simulink model "state_feedback_simulink"  (R2015b)
settings: Solver=ode3  StartTime=0.0  StopTime=10  FixedStep=0.01  RelTol=1e-3
values from neighbouring files (symbols this model uses):
  K = place(A,B,P)    [drone_config.m]
libraries: aerolib6dof2 x1
settings Model: Creator=rcasado  LastModifiedBy=rcasado
settings DataIOCC: SaveFormat=Array
settings DebuggingCC: MultiTaskRateTransMsg=warning
settings HardwareCC: ProdBitPerPointer=32  ProdLargestAtomicFloat=None  ProdIntDivRoundTo=Undefined  ProdEndianess=Unspecified  ProdWordSize=32  ProdHWDeviceType=32-bit Generic
settings GRTTargetCC: GeneratePreprocessorConditionals=Disable all
settings ConfigComp: CovModelRefEnable=Off

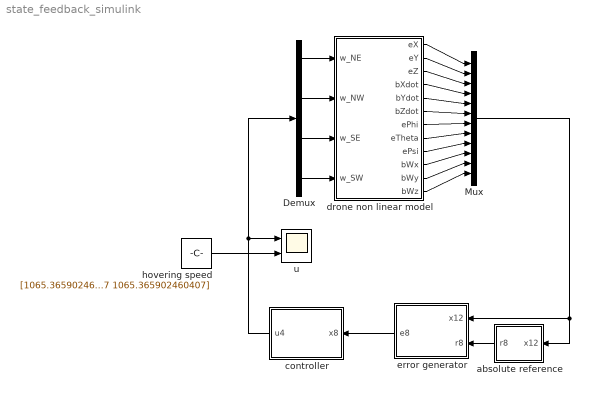
== system state_feedback_simulink ==
  Demux : Demux
  Mux : Mux  Inputs=12
  absolute reference : Subsystem
  controller : Subsystem
  drone non linear model : Subsystem
  error generator : Subsystem
  hovering speed : Constant  Value=[1065.365902460407 1065.365902460407 1065.365902460407 1065.365902460407]
  u : Scope  NumInputPorts=2
  wires:
  drone non linear model/1(eX) -> Mux/1
  drone non linear model/3(eZ) -> Mux/3
  drone non linear model/2(eY) -> Mux/2
  Demux/1 -> drone non linear model/1(w_NE)
  Demux/2 -> drone non linear model/2(w_NW)
  Demux/3 -> drone non linear model/3(w_SE)
  Demux/4 -> drone non linear model/4(w_SW)
  drone non linear model/12(bWz) -> Mux/12
  drone non linear model/11(bWy) -> Mux/11
  drone non linear model/4(bXdot) -> Mux/4
  drone non linear model/5(bYdot) -> Mux/5
  drone non linear model/6(bZdot) -> Mux/6
  drone non linear model/7(ePhi) -> Mux/7
  drone non linear model/8(eTheta) -> Mux/8
  drone non linear model/9(ePsi) -> Mux/9
  drone non linear model/10(bWx) -> Mux/10
  hovering speed/1 -> u/2
  Mux/1 -> absolute reference/1(x12), error generator/1(x12)
  error generator/1(e8) -> controller/1(x8)
  absolute reference/1(r8) -> error generator/2(r8)
  controller/1(u4) -> Demux/1, u/1

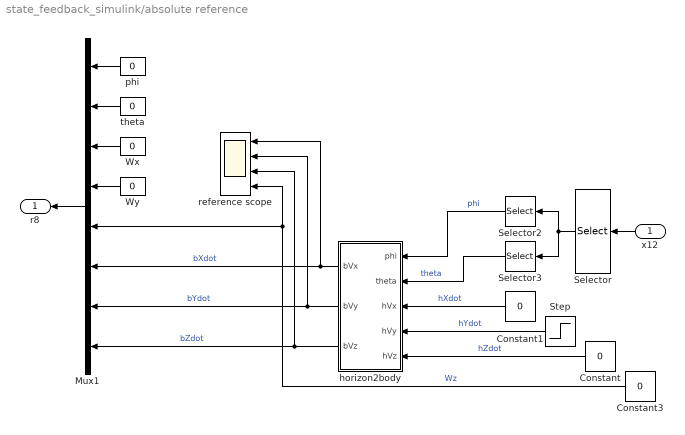
== system state_feedback_simulink/absolute reference ==
  x12 : Inport
  Constant : Constant  Value=0
  Constant1 : Constant  Value=0
  Constant3 : Constant  Value=0
  Mux1 : Mux  Inputs=8
  Selector : Selector  InputPortWidth=12  IndexOptions=Index vector (dialog)  Indices=[7,8]  OutputSizes=1
  Selector2 : Selector  InputPortWidth=2  IndexOptions=Index vector (dialog)  Indices=[1]  OutputSizes=1
  Selector3 : Selector  InputPortWidth=2  IndexOptions=Index vector (dialog)  Indices=[2]  OutputSizes=1
  Step : Step  Time=2  After=2  SampleTime=0
  Wx : Constant  Value=0
  Wy : Constant  Value=0
  horizon2body : Subsystem
  phi : Constant  Value=0
  reference scope : Scope  NumInputPorts=4
  theta : Constant  Value=0
  r8 : Outport
  wires:
  Step/1 -> horizon2body/4(hVy)  "hYdot"
  Constant1/1 -> horizon2body/3(hVx)  "hXdot"
  Constant3/1 -> Mux1/5, reference scope/4  "Wz"
  Constant/1 -> horizon2body/5(hVz)  "hZdot"
  Selector2/1 -> horizon2body/1(phi)  "phi"
  Selector3/1 -> horizon2body/2(theta)  "theta"
  x12/1 -> Selector/1
  Selector/1 -> Selector2/1, Selector3/1
  Mux1/1 -> r8/1
  Wx/1 -> Mux1/3
  Wy/1 -> Mux1/4
  horizon2body/1(bVx) -> reference scope/1, Mux1/6  "bXdot"
  horizon2body/3(bVz) -> Mux1/8, reference scope/3  "bZdot"
  horizon2body/2(bVy) -> reference scope/2, Mux1/7  "bYdot"
  phi/1 -> Mux1/1
  theta/1 -> Mux1/2

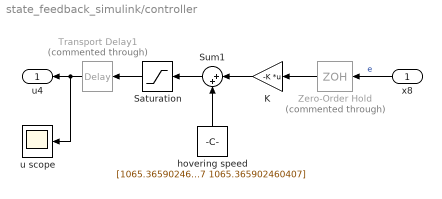
== system state_feedback_simulink/controller ==
  x8 : Inport
  K : Gain  Gain=-K  Multiplication=Matrix(K*u)
  Saturation : Saturate  UpperLimit=1650  LowerLimit=0
  Sum1 : Sum  Inputs=|++
  Transport Delay1 : TransportDelay  Commented=through  DelayTime=0.05
  Zero-Order Hold : ZeroOrderHold  Commented=through  SampleTime=0.01
  hovering speed : Constant  Value=[1065.365902460407 1065.365902460407 1065.365902460407 1065.365902460407]
  u scope : Scope
  u4 : Outport
  wires:
  Saturation/1 -> Transport Delay1/1
  K/1 -> Sum1/1
  x8/1 -> Zero-Order Hold/1  "e"
  hovering speed/1 -> Sum1/2
  Sum1/1 -> Saturation/1
  Zero-Order Hold/1 -> K/1
  Transport Delay1/1 -> u scope/1, u4/1

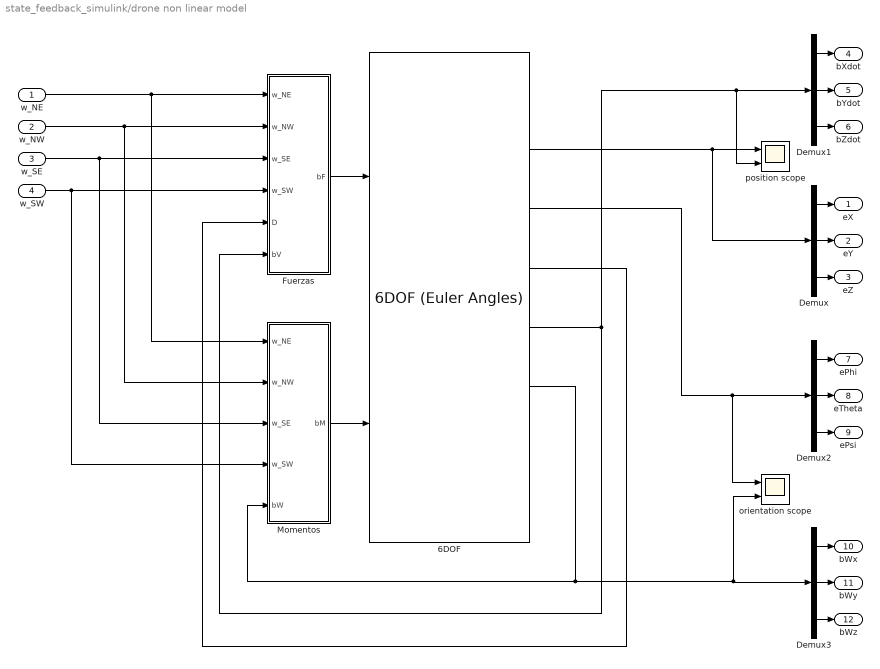
== system state_feedback_simulink/drone non linear model ==
  w_NE : Inport
  w_NW : Inport  Port=2
  w_SE : Inport  Port=3
  w_SW : Inport  Port=4
  6DOF : aerolib6dof2/6DOF (Euler Angles)  units=Metric (MKS)  mtype=Fixed  rep=Euler Angles  xme_0=[0 0 10]  Vm_0=[0 0 0]  eul_0=[0 0 deg2rad(0)]  pm_0=[0 0 0]  mass_0=1.840  mass_e=0.5  mass_f=2.0  inertia="[0.024916667  0  0 ; 0 0.024916667 0 ; 0 0 0.049066667]"  inertia_e=eye(3)  inertia_f=2*eye(3)  k_quat=1.0  vre_flag=on
  Demux{,1..3} (4 alike) : Demux  Outputs=3
  Fuerzas : Subsystem
  Momentos : Subsystem
  orientation scope : Scope  NumInputPorts=2
  position scope : Scope  NumInputPorts=2
  eX : Outport
  eY : Outport  Port=2
  eZ : Outport  Port=3
  bXdot : Outport  Port=4
  bYdot : Outport  Port=5
  bZdot : Outport  Port=6
  ePhi : Outport  Port=7
  eTheta : Outport  Port=8
  ePsi : Outport  Port=9
  bWx : Outport  Port=10
  bWy : Outport  Port=11
  bWz : Outport  Port=12
  wires:
  6DOF/2 -> Demux/1, position scope/1
  Momentos/1(bM) -> 6DOF/2
  w_NE/1 -> Momentos/1(w_NE), Fuerzas/1(w_NE)
  w_NW/1 -> Momentos/2(w_NW), Fuerzas/2(w_NW)
  w_SE/1 -> Momentos/3(w_SE), Fuerzas/3(w_SE)
  w_SW/1 -> Momentos/4(w_SW), Fuerzas/4(w_SW)
  6DOF/4 -> Fuerzas/5(D)
  Fuerzas/1(bF) -> 6DOF/1
  6DOF/6 -> Demux3/1, orientation scope/2, Momentos/5(bW)
  Demux/1 -> eX/1
  Demux/2 -> eY/1
  Demux/3 -> eZ/1
  6DOF/5 -> position scope/2, Demux1/1, Fuerzas/6(bV)
  Demux1/1 -> bXdot/1
  Demux1/2 -> bYdot/1
  Demux1/3 -> bZdot/1
  Demux2/1 -> ePhi/1
  Demux2/2 -> eTheta/1
  Demux2/3 -> ePsi/1
  Demux3/1 -> bWx/1
  Demux3/2 -> bWy/1
  Demux3/3 -> bWz/1
  6DOF/3 -> orientation scope/1, Demux2/1

== system state_feedback_simulink/error generator ==
  x12 : Inport
  r8 : Inport  Port=2
  Selector : Selector  InputPortWidth=12  IndexOptions=Index vector (dialog)  Indices=[7 8 10 11 12 4 5 6]  OutputSizes=1
  Sum : Sum  Inputs=|+-
  error scope : Scope
  estado scope : Scope
  referencia scope : Scope
  e8 : Outport
  wires:
  Sum/1 -> e8/1, error scope/1
  Selector/1 -> estado scope/1, Sum/1
  r8/1 -> Sum/2, referencia scope/1
  x12/1 -> Selector/1

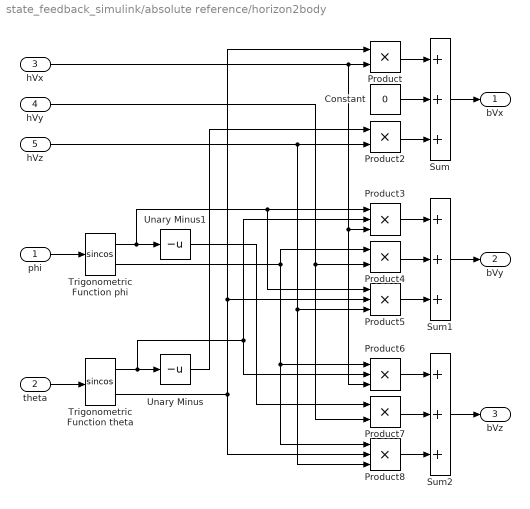
== system state_feedback_simulink/absolute reference/horizon2body ==
  phi : Inport
  theta : Inport  Port=2
  hVx : Inport  Port=3
  hVy : Inport  Port=4
  hVz : Inport  Port=5
  Constant : Constant  Value=0
  Product{,2,4,7} (4 alike) : Product
  Product{3,5..6,8} (4 alike) : Product  Inputs=3
  Sum : Sum  Inputs=3
  Sum1 : Sum  Inputs=3
  Sum2 : Sum  Inputs=3
  Trigonometric Function phi : Trigonometry  Operator=sincos
  Trigonometric Function theta : Trigonometry  Operator=sincos
  Unary Minus : UnaryMinus
  Unary Minus1 : UnaryMinus
  bVx : Outport
  bVy : Outport  Port=2
  bVz : Outport  Port=3
  wires:
  theta/1 -> Trigonometric Function theta/1
  phi/1 -> Trigonometric Function phi/1
  Trigonometric Function phi/2 -> Product4/1, Product8/1, Product6/1
  Trigonometric Function theta/2 -> Product8/2, Product/1, Product5/2
  Trigonometric Function theta/1 -> Product3/2, Product6/2, Unary Minus/1
  Trigonometric Function phi/1 -> Unary Minus1/1, Product5/1, Product3/1
  Sum/1 -> bVx/1
  Sum1/1 -> bVy/1
  Sum2/1 -> bVz/1
  Product/1 -> Sum/1
  Constant/1 -> Sum/2
  Product2/1 -> Sum/3
  Product3/1 -> Sum1/1
  Product4/1 -> Sum1/2
  Product5/1 -> Sum1/3
  Product6/1 -> Sum2/1
  Product7/1 -> Sum2/2
  Product8/1 -> Sum2/3
  hVx/1 -> Product6/3, Product3/3, Product/2
  hVy/1 -> Product7/2, Product4/2
  hVz/1 -> Product8/3, Product5/3, Product2/2
  Unary Minus/1 -> Product2/1
  Unary Minus1/1 -> Product7/1

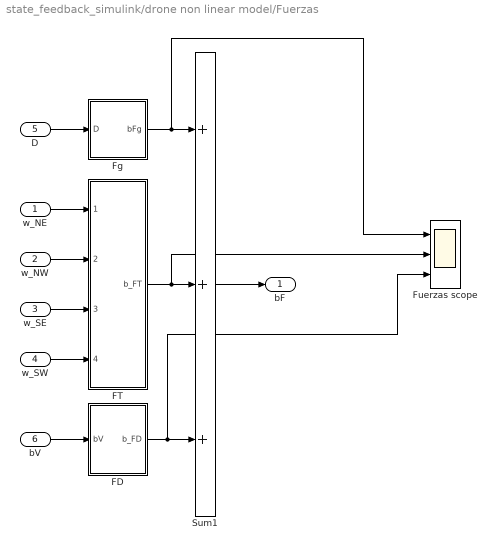
== system state_feedback_simulink/drone non linear model/Fuerzas ==
  w_NE : Inport
  w_NW : Inport  Port=2
  w_SE : Inport  Port=3
  w_SW : Inport  Port=4
  D : Inport  Port=5
  bV : Inport  Port=6
  FD : Subsystem
  FT : Subsystem
  Fg : Subsystem
  Fuerzas scope : Scope  NumInputPorts=3
  Sum1 : Sum  Inputs=+++
  bF : Outport
  wires:
  D/1 -> Fg/1(D)
  Fg/1(bFg) -> Fuerzas scope/1, Sum1/1
  FT/1(b_FT) -> Fuerzas scope/2, Sum1/2
  w_SW/1 -> FT/4(w_SW)
  w_NE/1 -> FT/1(w_NE)
  w_SE/1 -> FT/3(w_SE)
  w_NW/1 -> FT/2(w_NW)
  Sum1/1 -> bF/1
  bV/1 -> FD/1(bV)
  FD/1(b_FD) -> Sum1/3, Fuerzas scope/3

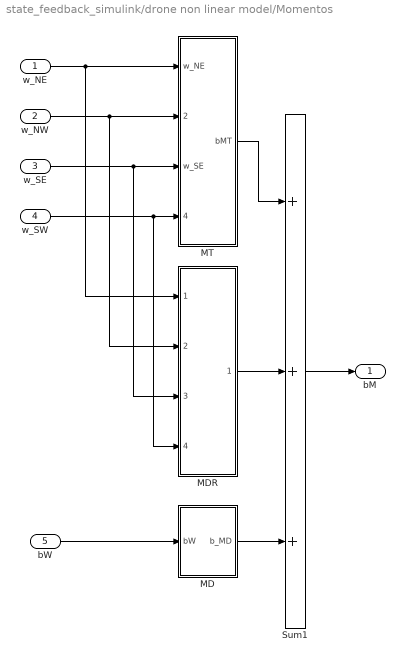
== system state_feedback_simulink/drone non linear model/Momentos ==
  w_NE : Inport
  w_NW : Inport  Port=2
  w_SE : Inport  Port=3
  w_SW : Inport  Port=4
  bW : Inport  Port=5
  MD : Subsystem
  MDR : Subsystem
  MT : Subsystem
  Sum1 : Sum  Inputs=+++
  bM : Outport
  wires:
  bW/1 -> MD/1(bW)
  MT/1(bMT) -> Sum1/1
  w_SW/1 -> MDR/4(w_SW), MT/4(w_SW)
  w_NE/1 -> MDR/1(w_NE), MT/1(w_NE)
  w_SE/1 -> MDR/3(w_SE), MT/3(w_SE)
  w_NW/1 -> MDR/2(w_NW), MT/2(w_NW)
  Sum1/1 -> bM/1
  MD/1(b_MD) -> Sum1/3
  MDR/1(b_MDR) -> Sum1/2

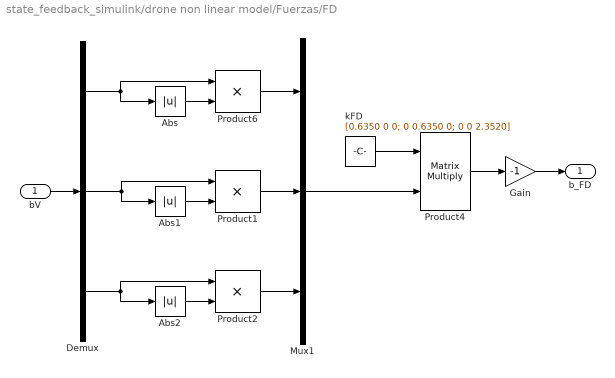
== system state_feedback_simulink/drone non linear model/Fuerzas/FD ==
  bV : Inport
  Abs : Abs
  Abs1 : Abs
  Abs2 : Abs
  Demux : Demux  Outputs=3
  Gain : Gain  Gain=-1
  Mux1 : Mux  Inputs=3
  Product1 : Product
  Product2 : Product
  Product4 : Product  Multiplication=Matrix(*)
  Product6 : Product
  kFD : Constant  Value=[0.6350 0 0; 0 0.6350 0; 0 0 2.3520]
  b_FD : Outport
  wires:
  kFD/1 -> Product4/1
  Product4/1 -> Gain/1
  Mux1/1 -> Product4/2
  Product1/1 -> Mux1/2
  bV/1 -> Demux/1
  Abs/1 -> Product6/2
  Abs1/1 -> Product1/2
  Abs2/1 -> Product2/2
  Demux/1 -> Product6/1, Abs/1
  Demux/2 -> Product1/1, Abs1/1
  Demux/3 -> Product2/1, Abs2/1
  Product6/1 -> Mux1/1
  Product2/1 -> Mux1/3
  Gain/1 -> b_FD/1

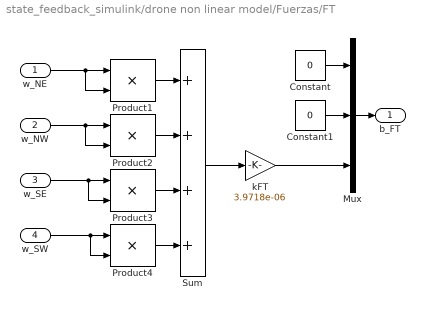
== system state_feedback_simulink/drone non linear model/Fuerzas/FT ==
  w_NE : Inport
  w_NW : Inport  Port=2
  w_SE : Inport  Port=3
  w_SW : Inport  Port=4
  Constant : Constant  Value=0
  Constant1 : Constant  Value=0
  Mux : Mux  Inputs=3
  Product{1..4} (4 alike) : Product
  Sum : Sum  Inputs=++++
  kFT : Gain  Gain=3.9718e-06
  b_FT : Outport
  wires:
  Product4/1 -> Sum/4
  Product3/1 -> Sum/3
  Product2/1 -> Sum/2
  w_NW/1 -> Product2/2, Product2/1
  w_NE/1 -> Product1/2, Product1/1
  Product1/1 -> Sum/1
  Mux/1 -> b_FT/1
  w_SE/1 -> Product3/2, Product3/1
  w_SW/1 -> Product4/2, Product4/1
  Sum/1 -> kFT/1
  Constant/1 -> Mux/1
  Constant1/1 -> Mux/2
  kFT/1 -> Mux/3

== system state_feedback_simulink/drone non linear model/Fuerzas/Fg ==
  D : Inport
  Fg scope : Scope  Commented=on  NumInputPorts=2
  Product : Product  Multiplication=Matrix(*)
  g : Gain  Gain=[0; 0; -9.8]
  masa : Constant  Value=1.840
  bFg : Outport
  wires:
  Product/1 -> Fg scope/2, bFg/1
  D/1 -> Product/1
  masa/1 -> g/1
  g/1 -> Fg scope/1, Product/2  "Fg"

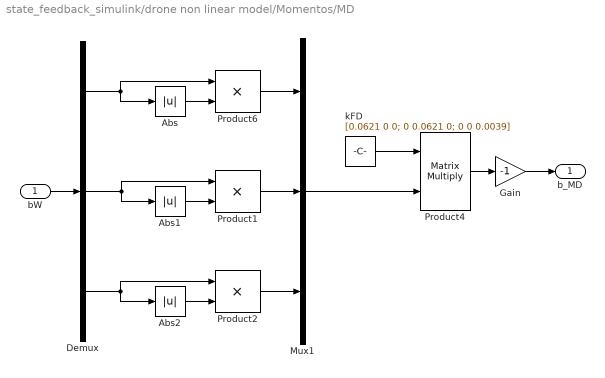
== system state_feedback_simulink/drone non linear model/Momentos/MD ==
  bW : Inport
  Abs : Abs
  Abs1 : Abs
  Abs2 : Abs
  Demux : Demux  Outputs=3
  Gain : Gain  Gain=-1
  Mux1 : Mux  Inputs=3
  Product1 : Product
  Product2 : Product
  Product4 : Product  Multiplication=Matrix(*)
  Product6 : Product
  kFD : Constant  Value=[0.0621 0 0; 0 0.0621 0; 0 0 0.0039]
  b_MD : Outport
  wires:
  kFD/1 -> Product4/1
  Product4/1 -> Gain/1
  Mux1/1 -> Product4/2
  Product1/1 -> Mux1/2
  bW/1 -> Demux/1
  Abs/1 -> Product6/2
  Abs1/1 -> Product1/2
  Abs2/1 -> Product2/2
  Demux/1 -> Product6/1, Abs/1
  Demux/2 -> Product1/1, Abs1/1
  Demux/3 -> Product2/1, Abs2/1
  Product6/1 -> Mux1/1
  Product2/1 -> Mux1/3
  Gain/1 -> b_MD/1

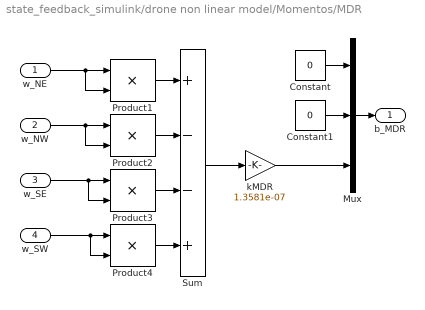
== system state_feedback_simulink/drone non linear model/Momentos/MDR ==
  w_NE : Inport
  w_NW : Inport  Port=2
  w_SE : Inport  Port=3
  w_SW : Inport  Port=4
  Constant : Constant  Value=0
  Constant1 : Constant  Value=0
  Mux : Mux  Inputs=3
  Product{1..4} (4 alike) : Product
  Sum : Sum  Inputs=+--+
  kMDR : Gain  Gain=1.3581e-07
  b_MDR : Outport
  wires:
  Product4/1 -> Sum/4
  Product3/1 -> Sum/3
  Product2/1 -> Sum/2
  w_NW/1 -> Product2/2, Product2/1
  w_NE/1 -> Product1/2, Product1/1
  Product1/1 -> Sum/1
  Mux/1 -> b_MDR/1
  w_SE/1 -> Product3/2, Product3/1
  w_SW/1 -> Product4/2, Product4/1
  Sum/1 -> kMDR/1
  Constant/1 -> Mux/1
  Constant1/1 -> Mux/2
  kMDR/1 -> Mux/3

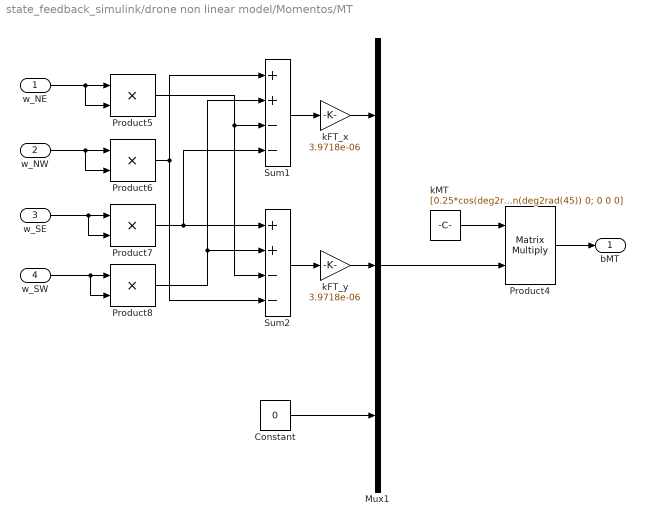
== system state_feedback_simulink/drone non linear model/Momentos/MT ==
  w_NE : Inport
  w_NW : Inport  Port=2
  w_SE : Inport  Port=3
  w_SW : Inport  Port=4
  Constant : Constant  Value=0
  Mux1 : Mux  Inputs=3
  Product4 : Product  Multiplication=Matrix(*)
  Product{5..8} (4 alike) : Product
  Sum1 : Sum  Inputs=++--
  Sum2 : Sum  Inputs=++--
  kFT_x : Gain  Gain=3.9718e-06
  kFT_y : Gain  Gain=3.9718e-06
  kMT : Constant  Value=[0.25*cos(deg2rad(45)) 0 0; 0 0.25*sin(deg2rad(45)) 0; 0 0 0]
  bMT : Outport
  wires:
  kMT/1 -> Product4/1
  Product4/1 -> bMT/1
  Product8/1 -> Sum1/2, Sum2/2
  Product7/1 -> Sum2/1, Sum1/4
  w_NW/1 -> Product6/2, Product6/1
  w_NE/1 -> Product5/2, Product5/1
  Product6/1 -> Sum2/4, Sum1/1
  Mux1/1 -> Product4/2
  w_SE/1 -> Product7/2, Product7/1
  w_SW/1 -> Product8/2, Product8/1
  kFT_y/1 -> Mux1/2
  Sum1/1 -> kFT_x/1
  Sum2/1 -> kFT_y/1
  Product5/1 -> Sum2/3, Sum1/3
  kFT_x/1 -> Mux1/1
  Constant/1 -> Mux1/3
